simulink model "m020_DynamicDeadZone"  (R2022a)
settings: Solver=VariableStepAuto  StartTime=0.0  StopTime=10.0  RelTol=1e-3
libraries: simulink x1
settings Model: Creator=Admin  LastModifiedBy=Admin

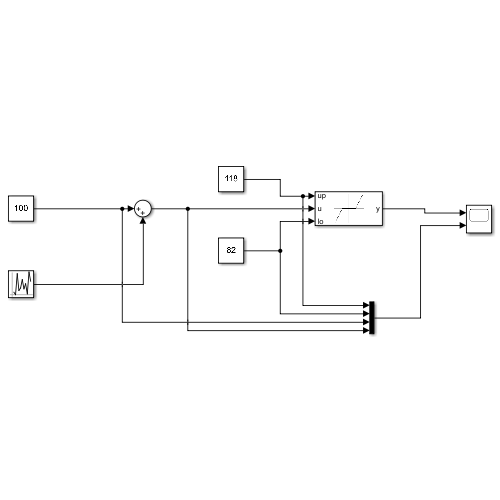
[thumbnail: Simulink's stored preview of the top-level diagram]
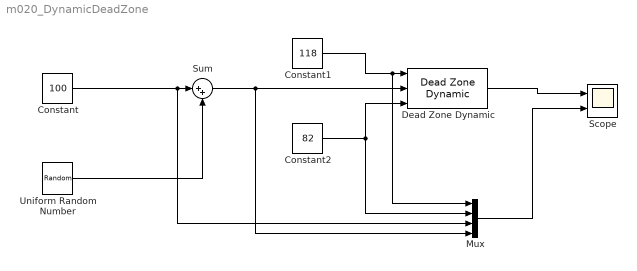
== system m020_DynamicDeadZone ==
  Constant : Constant  Value=100
  Constant1 : Constant  Value=118
  Constant2 : Constant  Value=82
  Dead Zone Dynamic : simulink/Discontinuities/Dead Zone Dynamic
      settings: SourceProductBaseCode=SL
  Mux : Mux
  Scope : Scope  NumInputPorts=2
  Sum : Sum  Inputs=|++
  Uniform Random Number : UniformRandomNumber  Minimum=-20  Maximum=20  SampleTime=0.02
  wires:
  Uniform Random Number/1 -> Sum/2
  Sum/1 -> Mux/4, Dead Zone Dynamic/2
  Dead Zone Dynamic/1 -> Scope/1
  Constant/1 -> Mux/3, Sum/1
  Mux/1 -> Scope/2
  Constant1/1 -> Mux/1, Dead Zone Dynamic/1
  Constant2/1 -> Mux/2, Dead Zone Dynamic/3
